simulink model "hcu_main_dspace"  (Simulink 8.2)
settings: Solver=FixedStepDiscrete  StartTime=0.0  StopTime=Inf  FixedStep=0.005  RelTol=1e-3
PostLoadFcn:
  | , if any(exist('dsrtsu_mdlpostloadfcn', 'file') == [2, 3, 6]), try dsrtsu_mdlpostloadfcn('Execute', bdroot); catch fprintf('Error in PostLoadFcn (dsrtsu_mdlpostloadfcn) for model "%s":\n %s\n', bdroot, lasterr); end, end,
values from neighbouring files (symbols this model uses):
  C_TASK_5MS_S = (	C_TICK_TIME_S      	)    [hcu_local_hdr.m]
  ENUM_GEARPOSN_1ST = uint8(  1  )    [hcu_local_hdr.m]
  ENUM_GEARPOSN_2ND = uint8(  2  )    [hcu_local_hdr.m]
  ENUM_GEARPOSN_3RD = uint8(  3  )    [hcu_local_hdr.m]
  ENUM_GEARPOSN_4TH = uint8(  4  )    [hcu_local_hdr.m]
  ENUM_GEARPOSN_5TH = uint8(  5  )    [hcu_local_hdr.m]
  ENUM_GEARPOSN_6TH = uint8(  6  )    [hcu_local_hdr.m]
  ENUM_GEARPOSN_R = uint8(  7  )    [hcu_local_hdr.m]
undefined symbols (not defined in the file or in its folder): rticanmm_blockfcn, rticanmm_initfcn
libraries: rtimmsu_dsrtlib x3, simulink x2, hal x2, app x1, rtiethernetudplib x1, inp x1, outp x1, hcu_lib x1
(part 1 of 4)
settings Model: DSRTSU_INTERNAL_RTI_VER=440  DSRTSU_INTERNAL_RTI_TYPE=rti1401  RTICANMMDATA=struct('GeneralSetupData',struct('modelroot','D:\ActiveSafetyDepartment\SVN\trunk\ADAS_Softwares\HTDragon\software\sw_development\arch','generalsettings',struct('filesettings',struct('destfolder',struct('Name','..\build\RTICANMM_FILES','Check',1),'buildfolder',struct('Name','.','Check',1),'AbsDestfolder',struct('Name','D:\ActiveSafetyDepartment\SVN\trunk\ADAS_Softwares\HTDragon\software\sw_development\build\RTICANMM_FILES'),'AbsBuildfolder',struct('Name','D:\ActiveSafetyDepartment\SVN\trunk\ADAS_Softwares\HTDragon\software\sw_development\arch'))),'options',struct('addpaths',1,'rmpaths',1,'addtrcexclusion',1,'cannavigator',struct('checkmonitoring',1),'show_usrtrc',0,'use_usrtrc',0,'addpath2usrmk',1),'advanced',struct('options',[1 1 1 1 1 1 1 1 1 1 1 1 1 1 1 1 1 1 1 1 1 1 1 1 1 1 1 1 1 1 1 1 1 1 1 1 1 1 1 1 1 1 1 1 1 1 1 1 1 1 1 1 1 1 1 1 1 1 1 1 1 1 1 1 1 1 1 1 1 1 1 1 1 1 1 1 1 1 1 1 1 1 1 1 1 1 1 1 1 1 1 1 1 1 1 1 1 1 1 1]),'MPSetup',{{}},'modelname','hcu_main_dspace','blockdata',struct('generalsettings',struct('filesettings',struct('destfolder',struct('Name','.','Check',1),'AbsDestfolder',struct('Name','T:\TOOL_SOURCES\CANnedy\m'),'buildfolder',struct('Name','.','Check',1),'AbsBuildfolder',struct('Name','C:\MATLAB6p5\work'))),'options',struct('addpaths',1,'rmpaths',1,'addpath2usrmk',1),'modelname','rticanmmlib','modelroot','T:\TOOL_SOURCES\CANnedy\m'),'MMType','RTICANMM','block',['hcu_main_dspace/RTICANMM' char(10) 'GeneralSetup'],'userdata',struct('HostServiceChannelID',{{'CAN_2',[],'CAN_1'}}),'RTI',struct('Type','RTI1401','Ver','7.2','Date','02-May-2014'),'version','3.0.735671.4434490741'))  DSRTSU_INTERNAL_RTIFPGA=30  Creator=11116  LastModifiedBy=14069  BufferReuse=off
settings DataIOCC: SignalLoggingSaveFormat=Dataset
settings OptimizationCC: BlockReduction=off  OptimizeBlockIOStorage=off  BufferReuse=off  ExpressionFolding=off  ExpressionDepthLimit=128  LocalBlockOutputs=off
settings DebuggingCC: CheckSSInitialOutputMsg=off  FcnCallInpInsideContextMsg=EnableAllAsError  StateNameClashWarn=none
settings HardwareCC: ProdIntDivRoundTo=Zero  ProdEndianess=BigEndian  ProdHWDeviceType=Generic->Custom  TargetIntDivRoundTo=Zero  TargetEndianess=BigEndian  TargetHWDeviceType=Generic->Custom
settings RTWCC: SystemTargetFile=rti1401.tlc  MakeCommand=make_rti  TemplateMakefile=rti1401.tmf  Description=dSPACE DS1401 Hardware Platform  ProcessScript=rti1401_make_rtw_hook
settings STFCustomTargetCC: CodeReplacementLibrary=ANSI_C  ParMdlRefBuildCompliant=on  GeneratePreprocessorConditionals=Disable all  SystemTargetFile=rti1401.tlc
settings GRTTargetCC: CompOptLevelCompliant=off  ConcurrentExecutionCompliant=off  MatFileLogging=off  ExtModeMexFile=noextcomm
settings CustomProperty: DataType=RTWOptions_EnumType_C__Program Files (x86)_dSPACE RCPHIL 2014-A_MATLAB_RTI_RTI1401_TLC_rti1401_1InitialSimState  Value=RUN
settings EnumStrPairs: String=RUN

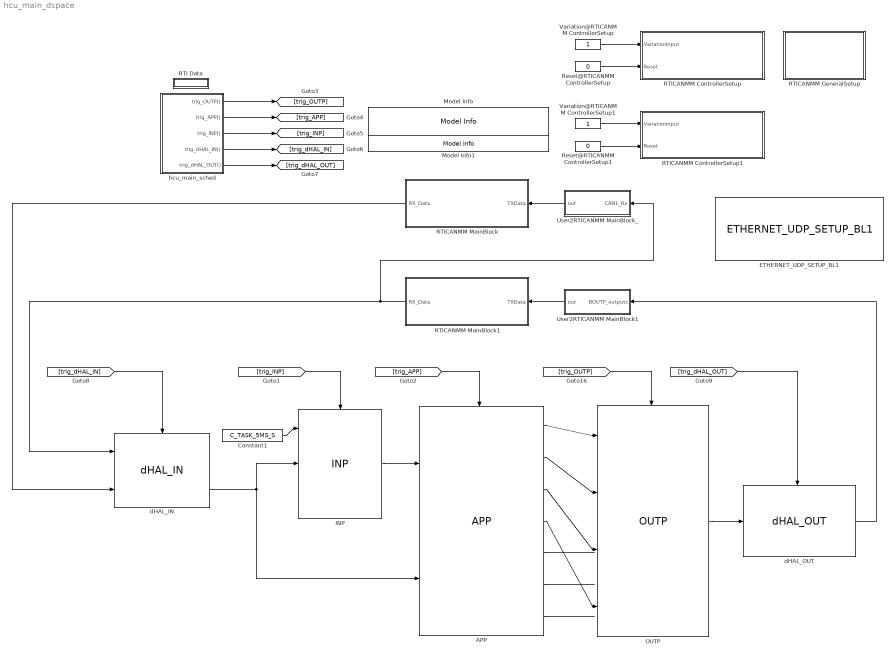
== system hcu_main_dspace ==
  APP : app/APP
  Constant1 : Constant  Value=C_TASK_5MS_S  OutDataTypeStr=single
  ETHERNET_UDP_SETUP_BL1 : rtiethernetudplib/ETHERNET_UDP_SETUP_BL1  DSProperties=struct('RTI',struct('Version',uint32(1),'BlockType',struct('isSLSource',uint8(0),'isSLSink',uint8(0),'isHWSource',uint8(0),'isHWSink',uint8(0),'isSetup',uint8(0),'isInline',uint8(1),'isNonInline',uint8(1),'isInterrupt',uint8(0),'isChannelwise',uint8(0)),'IOBoardType','DSETHERNETUDP','UnitType','ETHUDP','Identifier','SETUP','DialogType','ML','BlockSet','RTIETHERNETUDP','SlaveProcessor','NONE'))  RTIBlockInterface=struct('OutputPortsActive',0,'OutputPortsWidth',int32(1),'DialogFcn','rtiethernetudpsetupgui','InitLevel',3,'BlockDisplay',{{['Ethernet UDP Setup\nInterface Name: rti_ethernet_interface_name\nBoard Type: ETH Type 1\nModule: 1\nLocal IP Address: 192.168.140.11'],'center'}},'IconTransparency','on','BlockName',struct('Token',{{'ETHERNET_UDP_SETUP_BL1'}}))  RTIBlockParameters=struct('BoardType',{{1,'OFF',[]}},'ModuleNo',{{1,'ON',[1 16]}},'ChannelNo',{{1,'ON',[1 2]}},'InterfaceName',{{'rti_ethernet_interface_name','OFF',[]}},'LocalIpAddress',{{'192.168.140.11','OFF',[]}},'EnableSocket1',{{1,'OFF',[0 1]}},'LocalPortSocket1',{{'30000','OFF',[0 65535]}},'RemoteIpAddrSocket1',{{'192.168.140.10','OFF',[]}},'RemotePortSocket1',{{'30000','OFF',[0 65535]}},'EnableSocket2',{{1,'OFF',[0 1]}},'LocalPortSocket2',{{'30000','OFF',[0 65535]}},'RemoteIpAddrSocket2',{{'0.0.0.0','OFF',[]}},'RemotePortSocket2',{{'0','OFF',[0 65535]}},'EnableSocket3',{{0,'OFF',[0 1]}},'LocalPortSocket3',{{'5002','OFF',[0 65535]}},'RemoteIpAddrSocket3',{{'XXX.XXX.XXX.XXX','OFF',[]}},'RemotePortSocket3',{{'5002','OFF',[0 65535]}},'EnableSocket4',{{0,'OFF',[0 1]}},'LocalPortSocket4',{{'5003','OFF',[0 65535]}},'RemoteIpAddrSocket4',{{'XXX.XXX.XXX.XXX','OFF',[]}},'RemotePortSocket4',{{'5003','OFF',[0 65535]}},'LocalIpAddrHex',{{3232271371,'OFF',[]}},'RemoteIpAddrSocket1Hex',{{3232271370,'OFF',[]}},'RemoteIpAddrSocket2Hex',{{0,'OFF',[]}},'RemoteIpAddrSocket3Hex',{{0,'OFF',[]}},'RemoteIpAddrSocket4Hex',{{0,'OFF',[]}})  RTISFcnParameters=struct('BoardType','double','ModuleNo','double','ChannelNo','double','InterfaceName','char','LocalIpAddress','char','EnableSocket1','double','LocalPortSocket1','double','RemoteIpAddrSocket1','char','RemotePortSocket1','double','EnableSocket2','double','LocalPortSocket2','double','RemoteIpAddrSocket2','char','RemotePortSocket2','double','EnableSocket3','double','LocalPortSocket3','double','RemoteIpAddrSocket3','char','RemotePortSocket3','double','EnableSocket4','double','LocalPortSocket4','double','RemoteIpAddrSocket4','char','RemotePortSocket4','double','LocalIpAddrHex','double','RemoteIpAddrSocket1Hex','double','RemoteIpAddrSocket2Hex','double','RemoteIpAddrSocket3Hex','double','RemoteIpAddrSocket4Hex','double')  RTIBlockParaDefault=struct('BoardType',1,'ModuleNo',1,'ChannelNo',1,'InterfaceName','rti_ethernet_interface_name','LocalIpAddress','XXX.XXX.XXX.XXX','EnableSocket1',0,'LocalPortSocket1',5000,'RemoteIpAddrSocket1','XXX.XXX.XXX.XXX','RemotePortSocket1',5000,'EnableSocket2',0,'LocalPortSocket2',5001,'RemoteIpAddrSocket2','XXX.XXX.XXX.XXX','RemotePortSocket2',5001,'EnableSocket3',0,'LocalPortSocket3',5002,'RemoteIpAddrSocket3','XXX.XXX.XXX.XXX','RemotePortSocket3',5002,'EnableSocket4',0,'LocalPortSocket4',5003,'RemoteIpAddrSocket4','XXX.XXX.XXX.XXX','RemotePortSocket4',5003,'LocalIpAddrHex',0,'RemoteIpAddrSocket1Hex',0,'RemoteIpAddrSocket2Hex',0,'RemoteIpAddrSocket3Hex',0,'RemoteIpAddrSocket4Hex',0)
  INP : inp/INP
  Model Info : simulink/Model-Wide Utilities/Model Info  InitialBlockCM=None  BlockCM=None  Frame=off  DisplayStringWithTags=%<ModelName>  HorizontalTextAlignment=Center  LeftAlignmentValue=0.5  SourceBlockDiagram=hcu_main_dspace  TagMaxNumber=20
  Model Info1 : simulink/Model-Wide Utilities/Model Info  InitialBlockCM=None  BlockCM=None  Frame=off  DisplayStringWithTags=$Id: ADAS_Test.slx 244 2013-12-20 03:05:12Z JuneXmas $  HorizontalTextAlignment=Center  LeftAlignmentValue=0.5  SourceBlockDiagram=hcu_main_dspace  TagMaxNumber=20
  OUTP : outp/OUTP
  RTI Data : Subsystem  Tag=struct('RTIDataServer',struct('RTIDataServerVs','2','RTIModelDescription','struct(''main'',''hcu_main_dspace'',''sub'','''',''isMp'',0)'))  LoadFcn="if exist('rtidc'), try,  rtidc('DataHostBlockClbLoad', gcbh); catch, disp(['Warning: ''LoadFcn'' for RTI Data block failed: ' lasterr]); end, end,"  mask(RTI_DATA_HOST){}
      mask help:
      | RTI Data Block.
      | This block is used by RTI to store internal model-dependent data.
      | Please keep this block on the root level of the model. Deleting this block will result in data loss.
      |
      | NEVER DELETE OR COPY THIS BLOCK!
      settings: CopyFcn="if exist('rtidc'), try,  rtidc('DataHostBlockClbCopy', gcbh); catch, disp(['Warning: ''CopyFcn'' for RTI Data block failed: ' lasterr]); end, end,"  DeleteFcn="if exist('rtidc'), try,  rtidc('DataHostBlockClbDelete', gcbh); catch, disp(['Warning: ''DeleteFcn'' for RTI Data block failed: ' lasterr]); end, end,"  ModelCloseFcn="if exist('rtidc'), try,  rtidc('DataHostBlockClbModelClose', gcbh); catch, disp(['Warning: ''ModelCloseFcn'' for RTI Data block failed: ' lasterr]); end, end,"  PreSaveFcn="if exist('rtidc'), try,  rtidc('DataHostBlockClbPreSave', gcbh); catch, disp(['Warning: ''PreSaveFcn'' for RTI Data block failed: ' lasterr]); end, end,"  PostSaveFcn="if exist('rtidc'), try,  rtidc('DataHostBlockClbPostSave', gcbh); catch, disp(['Warning: ''PostSaveFcn'' for RTI Data block failed: ' lasterr]); end, end,"  NameChangeFcn="if exist('rtidc'), try,  rtidc('DataHostBlockClbNameChange', gcbh); catch, disp(['Warning: ''NameChangeFcn'' for RTI Data block failed: ' lasterr]); end, end,"
      mask Help:
      | RTI Data Block.
      | This block is used by RTI to store internal model-dependent data.
      | Please keep this block on the root level of the model. Deleting this block will result in data loss.
      | 
      | NEVER DELETE OR COPY THIS BLOCK!
      mask Display:
      | text(0.5, 0.5, 'RTI Data', 'HorizontalAlignment', 'center');
      | plot([1 0]);
  RTICANMM ControllerSetup : Subsystem  InitFcn=rticanmm_blockfcn('InitFcn', 'CANnedySetup', gcb)  ClipboardFcn=rticanmm_blockfcn('ClipboardFcn', 'CANnedySetup', gcb)  mask(RTICANMM){DSProperties=struct('RTI',struct('Version',uint32(1),'BlockType',struct('isSLSource',uint8(1),'isSLSink',uint8(1),'isHWSource',uint8(0),'isHWSink',uint8(0),'isSetup',uint8(0),'isInline',uint8(1),'isNonInline',uint8(0),'isInterrupt',uint8(0),'isChannelwise',uint8(0)),'IOBoardType','RTICANMM','UnitType','RTICANMM','Identifier','BUSSETUP','DialogType','SL','BlockSet','RTICANMM','SlaveProcessor','CAN')), CANMMProperties=struct('cannedy',struct('data',struct('options',struct('controllername','CAN_1','controllernameautomatic',[],'loglevel','0','checkrealtime',0,'checkchangebaudrate',0,'sampletime','1.000','CANControllerStatus',0,'NumberofStuffErr',0,'NumberofFormErr',0,'NumberofAckErr',0,'NumberofBit0Err',0,'NumberofsuccrecRX',0,'Numberofsuccsent',0,'NumberofBit1Err',0,'NumberofCRCErr',0,'NumberoflostRX',0,'Busoff',0,'Busload',0,'OperationPending',0,'TxRetryCount',3,'addtrcexclusion',logical(1),'cannavigator',struct('checkmonitoring',0,'checkinternmonitoring',0),'show_usrtrc',0,'use_usrtrc',0),'modelroot','D:\ADAS\ADAS\trunk\Demo\AI\ACM_d2','generalsettings',struct('setupdata',struct('board',['CAN Type 1'],'boardno',1,'channelno',1,'Type','STD','transceiver','ISO11898-2','busconfig','0x0','feedthrough','false','resistance',struct('r120',0,'roff',1,'r16',1,'r10',0),'baudrate','500','Frequency',[24 36],'samplemode',1,'commChannelTJA1041',6,'config',struct('standard',1,'advanced',0,'register',struct('btr0','0xC0','btr1','0x6F','sp','70','sjw','3','tseg1','15','tseg2','6','brp','0','smpl','0','btr0_36','0x41','btr1_36','0x1E','sp_36','88','sjw_36','1','tseg1_36','14','tseg2_36','1','brp_36','1','smpl_36','0','btr0_64','0x43','btr1_64','0x1C','sp_64','87','sjw_64','1','tseg1_64','12','tseg2_64','1','brp_64','3','smpl_64','0')),'channelcfg',struct('INTENDISABLE','CAN_INT_DISABLE','intenable',0),'SETUPID','RTICANMM_CAN_1_ID','CONTROLLER_ID','CANMM_CTL_SETUP_CAN_1','mainblock_includefile','RTICANMM_SETUP_CAN_1','termination','TERMINATION_OFF'),'filesettings',struct('destfolder',struct('Name','RTICANMM_FILES','Check',1),'buildfolder',struct('Name','.','Check',1))),'advanced',struct('options',[1 1 1 1 1 1 1 1 1 1 1 1 1 1 1 1 1 1 1 1 1 1 1 1 1 1 1 1 1 1 1 1 1 1 1 1 1 1 1 1 1 1 1 1 1 1 1 1 1 1 1 1 1 1 1 1 1 1 1 1 1 1 1 1 1 1 1 1 1 1 1 1 1 1 1 1 1 1 1 1 1 1 1 1 1 1 1 1 1 1 1 1 1 1 1 1 1 1 1 1]),'partialnetdata',struct('switchedon',0,'format','STD','idmask',['XXXXX XXXXXXXX XXXXXXXX XXXXXXXX'],'idcode','0','idfilter','0','datamaskused',0,'datalength','0','datamask','0x0000000000000000','partialnetworkenable',0)),'blk',['hcu_main_dspace/RTICANMM' char(10) 'ControllerSetup'],'allgeneratedfiles',{{'D:\ActiveSafetyDepartment\SVN\trunk\ADAS_Softwares\HTDragon\software\sw_development\build\RTICANMM_FILES\RTICANMM_SETUP_CAN_1.c','D:\ActiveSafetyDepartment\SVN\trunk\ADAS_Softwares\HTDragon\software\sw_development\build\RTICANMM_FILES\RTICANMM_SETUP_CAN_1.h','d:\activesafetydepartment\svn\trunk\adas_softwares\htdragon\software\sw_development\build\rticanmm_files\rticanmm_setup_can_1.mexw32'}},'ismp',logical(0),'BlockDataVersion','0.6.0','recreate',0,'CANnedyTag','EPAS'),'CANnedynew',0,'CANnedySettings','CAN_1','GeneratedFiles',{{'D:\ActiveSafetyDepartment\SVN\trunk\ADAS_Softwares\HTDragon\software\sw_development\build\RTICANMM_FILES\RTICANMM_SETUP_CAN_1.c','D:\ActiveSafetyDepartment\SVN\trunk\ADAS_Softwares\HTDragon\software\sw_development\build\RTICANMM_FILES\RTICANMM_SETUP_CAN_1.h','d:\activesafetydepartment\svn\trunk\adas_softwares\htdragon\software\sw_development\build\rticanmm_files\rticanmm_setup_can_1.mexw32'}},'SFCN','RTICANMM_SETUP_CAN_1.c','HostService',struct('Tags',struct('DATA','RTICANMM_MonitorData','Enable','CANMMMonitor_CAN_1','TimeStamp','MonitoringTimeStamp_CAN_1'),'DATA',struct('Length',4),'Info',struct('Desc',{'ID','Service','Data1','Data2'}),'Names',struct('Enable','Monitoring_Enable','TimeStamp','Monitoring_TimeStamp'),'ChannelID',3)), CANMMType=CANnedySetup, CANMMFolder=D:\ActiveSafetyDepartment\SVN\trunk\ADAS_Softwares\HTDragon\software\sw_development\arch, CANMMDestFolder=..\build\RTICANMM_FILES, CANMMSettings=CAN_1, CANMMSFcn=RTICANMM_SETUP_CAN_1, CANMMBoard=DS1401, CANMMBoardNum=1, CANMMChannel=1}
      settings: AttributesFormatString=%<CANMMSettings>: %<CANMMBoard>_B%<CANMMBoardNum>_C%<CANMMChannel>  CopyFcn=rticanmm_blockfcn('CopyFcn', 'CANnedySetup', gcb)  DeleteFcn=rticanmm_blockfcn('DeleteFcn', 'CANnedySetup', gcb)  ModelCloseFcn=rticanmm_blockfcn('ModelCloseFcn', 'CANnedySetup', gcb)  NameChangeFcn=rticanmm_blockfcn('NameChangeFcn', 'CANnedySetup', gcb)  OpenFcn=try, rticanmm_setup_gui('create',gcb); ; catch,errordlg({lasterr, '','Please check your RTI installation.'},['Error: ' upper(bdroot)], 'replace'); end  MoveFcn=rticanmm_blockfcn('MoveFcn', 'CANnedySetup', gcb)
      mask Help: eval('rticanmm_quickstart(''create'', gcb);', 'disp(lasterr);')
      mask Display:
      | disp('RTI CAN\nMultiMessage\nControllerSetup')
      | 
      | port_label('input', 1 , 'Variation')
      | port_label('input', 2 , 'Reset')
  RTICANMM ControllerSetup1 : Subsystem  InitFcn=rticanmm_blockfcn('InitFcn', 'CANnedySetup', gcb)  ClipboardFcn=rticanmm_blockfcn('ClipboardFcn', 'CANnedySetup', gcb)  mask(RTICANMM){DSProperties=struct('RTI',struct('Version',uint32(1),'BlockType',struct('isSLSource',uint8(1),'isSLSink',uint8(1),'isHWSource',uint8(0),'isHWSink',uint8(0),'isSetup',uint8(0),'isInline',uint8(1),'isNonInline',uint8(0),'isInterrupt',uint8(0),'isChannelwise',uint8(0)),'IOBoardType','RTICANMM','UnitType','RTICANMM','Identifier','BUSSETUP','DialogType','SL','BlockSet','RTICANMM','SlaveProcessor','CAN')), CANMMProperties=struct('cannedy',struct('data',struct('options',struct('controllername','CAN_2','controllernameautomatic',[],'loglevel','0','checkrealtime',0,'checkchangebaudrate',0,'sampletime','1.000','CANControllerStatus',0,'NumberofStuffErr',0,'NumberofFormErr',0,'NumberofAckErr',0,'NumberofBit0Err',0,'NumberofsuccrecRX',0,'Numberofsuccsent',0,'NumberofBit1Err',0,'NumberofCRCErr',0,'NumberoflostRX',0,'Busoff',0,'Busload',0,'OperationPending',0,'TxRetryCount',3,'addtrcexclusion',logical(1),'cannavigator',struct('checkmonitoring',0,'checkinternmonitoring',0),'show_usrtrc',0,'use_usrtrc',0),'modelroot','D:\ActiveSafetyDepartment\SVN\trunk\Demo\AI\ACM_d5','generalsettings',struct('setupdata',struct('board',['CAN Type 1'],'boardno',1,'channelno',2,'Type','STD','transceiver','ISO11898-2','busconfig','0x0','feedthrough','false','resistance',struct('r120',1,'roff',0,'r16',1,'r10',0),'baudrate','500','Frequency',[24 36],'samplemode',1,'commChannelTJA1041',6,'config',struct('standard',1,'advanced',0,'register',struct('btr0','0xC0','btr1','0x6F','sp','70','sjw','3','tseg1','15','tseg2','6','brp','0','smpl','0','btr0_36','0x41','btr1_36','0x1E','sp_36','88','sjw_36','1','tseg1_36','14','tseg2_36','1','brp_36','1','smpl_36','0','btr0_64','0x43','btr1_64','0x1C','sp_64','87','sjw_64','1','tseg1_64','12','tseg2_64','1','brp_64','3','smpl_64','0')),'channelcfg',struct('INTENDISABLE','CAN_INT_DISABLE','intenable',0),'SETUPID','RTICANMM_CAN_2_ID','CONTROLLER_ID','CANMM_CTL_SETUP_CAN_2','mainblock_includefile','RTICANMM_SETUP_CAN_2','termination','TERMINATION_ON'),'filesettings',struct('destfolder',struct('Name','RTICANMM_FILES','Check',1),'buildfolder',struct('Name','.','Check',1))),'advanced',struct('options',[1 1 1 1 1 1 1 1 1 1 1 1 1 1 1 1 1 1 1 1 1 1 1 1 1 1 1 1 1 1 1 1 1 1 1 1 1 1 1 1 1 1 1 1 1 1 1 1 1 1 1 1 1 1 1 1 1 1 1 1 1 1 1 1 1 1 1 1 1 1 1 1 1 1 1 1 1 1 1 1 1 1 1 1 1 1 1 1 1 1 1 1 1 1 1 1 1 1 1 1]),'partialnetdata',struct('switchedon',0,'format','STD','idmask',['XXXXX XXXXXXXX XXXXXXXX XXXXXXXX'],'idcode','0','idfilter','0','datamaskused',0,'datalength','0','datamask','0x0000000000000000','partialnetworkenable',0)),'blk',['hcu_main_dspace/RTICANMM' char(10) 'ControllerSetup1'],'allgeneratedfiles',{{'D:\ActiveSafetyDepartment\SVN\trunk\ADAS_Softwares\HTDragon\software\sw_development\build\RTICANMM_FILES\RTICANMM_SETUP_CAN_2.c','D:\ActiveSafetyDepartment\SVN\trunk\ADAS_Softwares\HTDragon\software\sw_development\build\RTICANMM_FILES\RTICANMM_SETUP_CAN_2.h','d:\activesafetydepartment\svn\trunk\adas_softwares\htdragon\software\sw_development\build\rticanmm_files\rticanmm_setup_can_2.mexw32'}},'ismp',logical(0),'BlockDataVersion','0.6.0','recreate',0,'CANnedyTag','TEST'),'CANnedynew',0,'CANnedySettings','CAN_2','GeneratedFiles',{{'D:\ActiveSafetyDepartment\SVN\trunk\ADAS_Softwares\HTDragon\software\sw_development\build\RTICANMM_FILES\RTICANMM_SETUP_CAN_2.c','D:\ActiveSafetyDepartment\SVN\trunk\ADAS_Softwares\HTDragon\software\sw_development\build\RTICANMM_FILES\RTICANMM_SETUP_CAN_2.h','d:\activesafetydepartment\svn\trunk\adas_softwares\htdragon\software\sw_development\build\rticanmm_files\rticanmm_setup_can_2.mexw32'}},'SFCN','RTICANMM_SETUP_CAN_2.c','HostService',struct('Tags',struct('DATA','RTICANMM_MonitorData','Enable','CANMMMonitor_CAN_2','TimeStamp','MonitoringTimeStamp_CAN_2'),'DATA',struct('Length',4),'Info',struct('Desc',{'ID','Service','Data1','Data2'}),'Names',struct('Enable','Monitoring_Enable','TimeStamp','Monitoring_TimeStamp'),'ChannelID',1)), CANMMType=CANnedySetup, CANMMFolder=D:\ActiveSafetyDepartment\SVN\trunk\ADAS_Softwares\HTDragon\software\sw_development\arch, CANMMDestFolder=..\build\RTICANMM_FILES, CANMMSettings=CAN_2, CANMMSFcn=RTICANMM_SETUP_CAN_2, CANMMBoard=DS1401, CANMMBoardNum=1, CANMMChannel=2}
      settings: AttributesFormatString=%<CANMMSettings>: %<CANMMBoard>_B%<CANMMBoardNum>_C%<CANMMChannel>  CopyFcn=rticanmm_blockfcn('CopyFcn', 'CANnedySetup', gcb)  DeleteFcn=rticanmm_blockfcn('DeleteFcn', 'CANnedySetup', gcb)  ModelCloseFcn=rticanmm_blockfcn('ModelCloseFcn', 'CANnedySetup', gcb)  NameChangeFcn=rticanmm_blockfcn('NameChangeFcn', 'CANnedySetup', gcb)  OpenFcn=try, rticanmm_setup_gui('create',gcb); ; catch,errordlg({lasterr, '','Please check your RTI installation.'},['Error: ' upper(bdroot)], 'replace'); end  MoveFcn=rticanmm_blockfcn('MoveFcn', 'CANnedySetup', gcb)
      mask Help: eval('rticanmm_quickstart(''create'', gcb);', 'disp(lasterr);')
      mask Display:
      | disp('RTI CAN\nMultiMessage\nControllerSetup')
      | 
      | port_label('input', 1 , 'Variation')
      | port_label('input', 2 , 'Reset')
  RTICANMM GeneralSetup : Subsystem  InitFcn=rticanmm_initfcn(gcb, 'CANnedySettings')  ClipboardFcn=rticanmm_blockfcn('ClipboardFcn', 'CANnedySettings', gcb)  mask(RTICANMM){DSProperties=struct('RTI',struct('Version',uint32(1),'BlockType',struct('isSLSource',uint8(1),'isSLSink',uint8(1),'isHWSource',uint8(0),'isHWSink',uint8(0),'isSetup',uint8(0),'isInline',uint8(1),'isNonInline',uint8(0),'isInterrupt',uint8(0),'isChannelwise',uint8(0)),'IOBoardType','RTICANMM','UnitType','RTICANMM','Identifier','GENERALSETUP','DialogType','SL','BlockSet','RTICANMM','SlaveProcessor','CAN')), CANMMDestFolder=..\build\RTICANMM_FILES, CANMMBuildDir=., CANMMAddPaths=on, CANMMAddpathUserMake=on, CANMMRemovePathOnclose=on, CANMMType=CANnedySettings, CANMMProperties=struct('modelroot','D:\ActiveSafetyDepartment\SVN\trunk\ADAS_Softwares\HTDragon\software\sw_development\arch','generalsettings',struct('filesettings',struct('destfolder',struct('Name','..\build\RTICANMM_FILES','Check',1),'buildfolder',struct('Name','.','Check',1),'AbsDestfolder',struct('Name','D:\ActiveSafetyDepartment\SVN\trunk\ADAS_Softwares\HTDragon\software\sw_development\build\RTICANMM_FILES'),'AbsBuildfolder',struct('Name','D:\ActiveSafetyDepartment\SVN\trunk\ADAS_Softwares\HTDragon\software\sw_development\arch'))),'options',struct('addpaths',1,'rmpaths',1,'addtrcexclusion',1,'cannavigator',struct('checkmonitoring',1),'show_usrtrc',0,'use_usrtrc',0,'addpath2usrmk',1),'advanced',struct('options',[1 1 1 1 1 1 1 1 1 1 1 1 1 1 1 1 1 1 1 1 1 1 1 1 1 1 1 1 1 1 1 1 1 1 1 1 1 1 1 1 1 1 1 1 1 1 1 1 1 1 1 1 1 1 1 1 1 1 1 1 1 1 1 1 1 1 1 1 1 1 1 1 1 1 1 1 1 1 1 1 1 1 1 1 1 1 1 1 1 1 1 1 1 1 1 1 1 1 1 1]),'MPSetup',{{}},'modelname','hcu_main_dspace','blockdata',struct('generalsettings',struct('filesettings',struct('destfolder',struct('Name','.','Check',1),'AbsDestfolder',struct('Name','T:\TOOL_SOURCES\CANnedy\m'),'buildfolder',struct('Name','.','Check',1),'AbsBuildfolder',struct('Name','C:\MATLAB6p5\work'))),'options',struct('addpaths',1,'rmpaths',1,'addpath2usrmk',1),'modelname','rticanmmlib','modelroot','T:\TOOL_SOURCES\CANnedy\m'),'MMType','RTICANMM','block',['hcu_main_dspace/RTICANMM' char(10) 'GeneralSetup'],'userdata',struct('HostServiceChannelID',{{'CAN_2',[],'CAN_1'}}),'RTI',struct('Type','RTI1401','Ver','7.2','Date','02-May-2014'),'version','3.0.735671.4434490741')}
      mask prompts: CANMMDestFolder "Destination Folder for generated Files:"; CANMMBuildDir "Build Directory (*_usr.mk, *_usr.trc)"; CANMMAddPaths "Add Paths automatically"; CANMMAddpathUserMake "Add Paths to UserMake-File"; CANMMRemovePathOnclose "Remove added Path on ModelClose"
      mask init:
      | rticanmm_initfcn(gcb,'CANnedyGeneralSettings')
      settings: CopyFcn=rticanmm_blockfcn('CopyFcn', 'CANnedySettings', gcb)  DeleteFcn=rticanmm_blockfcn('DeleteFcn', 'CANnedySettings', gcb)  ModelCloseFcn=rticanmm_blockfcn('CloseFcn', 'CANnedyGeneralSettings', gcb)  NameChangeFcn=rticanmm_blockfcn('NameChangeFcn', 'CANnedySettings', gcb)  OpenFcn=try, rticanmm_gs_gui('create',gcb), ; catch,errordlg({lasterr, '','Please check your RTI installation.'},['Error: ' upper(bdroot)], 'replace'); end  MoveFcn=rticanmm_blockfcn('MoveFcn', 'CANnedySettings', gcb)
      mask Help: eval('rticanmm_quickstart(''create'', gcb);', 'disp(lasterr);')
      mask Display: disp(sprintf(['RTI CAN\nMultiMessage\nGeneralSetup']))
  RTICANMM MainBlock : Subsystem  InitFcn=rticanmm_blockfcn('InitFcn', 'CANnedy', gcb)  ClipboardFcn=rticanmm_blockfcn('ClipboardFcn', 'CANnedy', gcb)  mask(RTICANMM){DSProperties=struct('RTI',struct('Version',uint32(1),'BlockType',struct('isSLSource',uint8(1),'isSLSink',uint8(1),'isHWSource',uint8(0),'isHWSink',uint8(0),'isSetup',uint8(0),'isInline',uint8(1),'isNonInline',uint8(0),'isInterrupt',uint8(0),'isChannelwise',uint8(0)),'IOBoardType','RTICANMM','UnitType','RTICANMM','Identifier','Mainblock','DialogType','SL','BlockSet','RTICANMM','SlaveProcessor','CAN')), CANMMProperties=struct('RTICANMMVersion','3.0','RTICANMMVersionIntern','3.0.735671.4434490741','RTICANMMDate','02-May-2014','Settings','RTICANMM_MAIN_CAN_2','UserTracePath','','ModelPath','D:\ActiveSafetyDepartment\SVN\trunk\ADAS_Softwares\HTDragon\software\sw_development\arch','filesettings',struct('FileName','..\..\..\..\CAN\IDIADA_CAN2_Chimo.dbc','IsRelative',1,'ClusterId',1,'ClusterList',{{'default'}},'destfolder',struct('Name','..\build\RTICANMM_FILES','Check',1),'buildfolder',struct('Name','.','Check',1),'onlyfreerawcapture',0,'overlapping2variant',0),'onlyfreerawcapture',0,'Board',['CAN Type 1'],'BoardNum','1','ChannelNum','2','Variation','1','SetupId','CAN_2','MARK',['2DBE3E4EF1BAADAF8427111C40D4CA';'085B5D53DE150542DA650E691DA8DD';'A43ABF07D72688DDE05877E4A4CD4F';'3C583CAA49F93CC5669B070848561E';'93657246D29663F85A60CA3CB29854'],'date','03-Dec-2015','clock',['03.12.2015 15:57:37'],'recreate',0,'RTIVER','RTI1401','j1939',0,'TRC',struct('include',1),'rtsupport',struct('XMLFile','D:\ActiveSafetyDepartment\SVN\trunk\ADAS_Softwares\HTDragon\software\sw_development\build\RTICANMM_FILES\RTICANMM_MAIN_CAN_2.xml','DBCXML',struct('Path','D:\ActiveSafetyDepartment\SVN\trunk\ADAS_Softwares\HTDragon\software\sw_development\build\RTICANMM_FILES\RTICANMM_MAIN_CAN_2_dbc.xml','support',1,'Name','IDIADA_CAN2_Chimo.dbc','Date',['15-十月-2015 11:52:08'],'Type','standard','DBCSupport','ON'))), CANMMType=CANnedy, CANMMUserTraceMerged=off, CANMMUserTracePath=, CANMMChannelNum=2, CANMMBoardNum=1, CANMMDestFolder=..\build\RTICANMM_FILES, CANMMFolder=., CANMMSetupId=CAN_2, CANMMsave2mat=['2DBE3E4EF1BAADAF8427111C40D4CA';'085B5D53DE150542DA650E691DA8DD';'A43ABF07D72688DDE05877E4A4CD4F';'3C583CAA49F93CC5669B070848561E';'93657246D29663F85A60CA3CB29854'], CANMMName=CAN_2, CANMMSettings=RTICANMM_MAIN_CAN_2, CANMMIntermediateTag=RTICANMM_MAIN_CAN_2_intermediate, CANMMsfcnname=RTICANMM_MAIN_CAN_2}
      mask init:
      | rticanmm_initfcn(gcb, CANMMType, CANMMsfcnname)
      settings: AttributesFormatString=CAN_2[CAN_2]: DS1401_B1_C2_V1  CopyFcn=rticanmm_blockfcn('CopyFcn', 'CANnedy', gcb)  DeleteFcn=rticanmm_blockfcn('DeleteFcn', 'CANnedy', gcb)  ModelCloseFcn=rticanmm_blockfcn('ModelCloseFcn', 'CANnedy', gcb)  NameChangeFcn=rticanmm_blockfcn('NameChangeFcn', 'CANnedy', gcb)  OpenFcn=try, rticanmm_main_gui('create',gcb); ; catch,errordlg({lasterr, '','Please check your RTI installation.'},['Error: ' upper(bdroot)], 'replace'); end  MoveFcn=rticanmm_blockfcn('MoveFcn', 'CANnedy', gcb)
      mask Help: eval('rticanmm_quickstart(''create'', gcb);', 'disp(lasterr);')
      mask Display:
      | disp(sprintf('RTI CAN\nMultiMessage\nMainSetup'))
      | port_label('input', 1, 'TX Data')
      | port_label('output', 1, 'RX Data')
  RTICANMM MainBlock1 : Subsystem  InitFcn=rticanmm_blockfcn('InitFcn', 'CANnedy', gcb)  ClipboardFcn=rticanmm_blockfcn('ClipboardFcn', 'CANnedy', gcb)  mask(RTICANMM){DSProperties=struct('RTI',struct('Version',uint32(1),'BlockType',struct('isSLSource',uint8(1),'isSLSink',uint8(1),'isHWSource',uint8(0),'isHWSink',uint8(0),'isSetup',uint8(0),'isInline',uint8(1),'isNonInline',uint8(0),'isInterrupt',uint8(0),'isChannelwise',uint8(0)),'IOBoardType','RTICANMM','UnitType','RTICANMM','Identifier','Mainblock','DialogType','SL','BlockSet','RTICANMM','SlaveProcessor','CAN')), CANMMProperties=struct('RTICANMMVersion','3.0','RTICANMMVersionIntern','3.0.735671.4434490741','RTICANMMDate','02-May-2014','Settings','RTICANMM_MAIN_CAN_1','UserTracePath','','ModelPath','D:\ActiveSafetyDepartment\SVN\trunk\ADAS_Softwares\HTDragon\software\sw_development\arch','filesettings',struct('FileName','..\..\..\..\CAN\ADAS_CAN1_Mule1_BSGEMS_MVCU_MEPS_20150610_db.dbc','IsRelative',1,'ClusterId',1,'ClusterList',{{'default'}},'destfolder',struct('Name','..\build\RTICANMM_FILES','Check',1),'buildfolder',struct('Name','.','Check',1),'onlyfreerawcapture',0,'overlapping2variant',0),'onlyfreerawcapture',0,'Board',['CAN Type 1'],'BoardNum','1','ChannelNum','1','Variation','1','SetupId','CAN_1','MARK',['472D3A1A3D5208B3D30AB78F04E268';'A50162927E39700EACAFCCF6AEEB36';'6294BC9383410CB3E84E79B296AFCF';'84400670336E8CD48E57496AA42E44';'1090534234403A3283605A55A13471'],'date','03-Dec-2015','clock',['03.12.2015 15:58:16'],'recreate',0,'RTIVER','RTI1401','j1939',0,'TRC',struct('include',1),'rtsupport',struct('XMLFile','D:\ActiveSafetyDepartment\SVN\trunk\ADAS_Softwares\HTDragon\software\sw_development\build\RTICANMM_FILES\RTICANMM_MAIN_CAN_1.xml','DBCXML',struct('Path','D:\ActiveSafetyDepartment\SVN\trunk\ADAS_Softwares\HTDragon\software\sw_development\build\RTICANMM_FILES\RTICANMM_MAIN_CAN_1_dbc.xml','support',1,'Name','ADAS_CAN1_Mule1_BSGEMS_MVCU_MEPS_20150610_db.dbc','Date',['12-十一月-2015 09:30:54'],'Type','standard','DBCSupport','ON'))), CANMMType=CANnedy, CANMMUserTraceMerged=off, CANMMUserTracePath=, CANMMChannelNum=1, CANMMBoardNum=1, CANMMDestFolder=..\build\RTICANMM_FILES, CANMMFolder=., CANMMSetupId=CAN_1, CANMMsave2mat=['472D3A1A3D5208B3D30AB78F04E268';'A50162927E39700EACAFCCF6AEEB36';'6294BC9383410CB3E84E79B296AFCF';'84400670336E8CD48E57496AA42E44';'1090534234403A3283605A55A13471'], CANMMName=CAN_1, CANMMSettings=RTICANMM_MAIN_CAN_1, CANMMIntermediateTag=RTICANMM_MAIN_CAN_1_intermediate, CANMMsfcnname=RTICANMM_MAIN_CAN_1}
      mask init:
      | rticanmm_initfcn(gcb, CANMMType, CANMMsfcnname)
      settings: AttributesFormatString=CAN_1[CAN_1]: DS1401_B1_C1_V1  CopyFcn=rticanmm_blockfcn('CopyFcn', 'CANnedy', gcb)  DeleteFcn=rticanmm_blockfcn('DeleteFcn', 'CANnedy', gcb)  ModelCloseFcn=rticanmm_blockfcn('ModelCloseFcn', 'CANnedy', gcb)  NameChangeFcn=rticanmm_blockfcn('NameChangeFcn', 'CANnedy', gcb)  OpenFcn=try, rticanmm_main_gui('create',gcb); ; catch,errordlg({lasterr, '','Please check your RTI installation.'},['Error: ' upper(bdroot)], 'replace'); end  MoveFcn=rticanmm_blockfcn('MoveFcn', 'CANnedy', gcb)
      mask Help: eval('rticanmm_quickstart(''create'', gcb);', 'disp(lasterr);')
      mask Display:
      | disp(sprintf('RTI CAN\nMultiMessage\nMainSetup'))
      | port_label('input', 1, 'TX Data')
      | port_label('output', 1, 'RX Data')
  Reset@RTICANMM ControllerSetup : Constant  Value=0  OutDataTypeStr=boolean
  Reset@RTICANMM ControllerSetup1 : Constant  Value=0  OutDataTypeStr=boolean
  User2RTICANMM MainBlock1 : Subsystem
      mask Display: disp('Mapping\nto RTICANMM')
  User2RTICANMM MainBlock_ : Subsystem
      mask Display: disp('Mapping\nto RTICANMM')
  Variation@RTICANMM ControllerSetup : Constant  OutDataTypeStr=uint8
  Variation@RTICANMM ControllerSetup1 : Constant  OutDataTypeStr=uint8
  dHAL_IN : hal/dHAL_IN
  dHAL_OUT : hal/dHAL_OUT
  hcu_main_sched : Stateflow chart  TreatAsAtomicUnit=on
  wires:
  Variation@RTICANMM ControllerSetup/1 -> RTICANMM ControllerSetup/1(VariationInput)
  Reset@RTICANMM ControllerSetup/1 -> RTICANMM ControllerSetup/2(Reset)
  Variation@RTICANMM ControllerSetup1/1 -> RTICANMM ControllerSetup1/1(VariationInput)
  Reset@RTICANMM ControllerSetup1/1 -> RTICANMM ControllerSetup1/2(Reset)
  hcu_main_sched/1(trig_OUTP()) -> [trig_OUTP]
  hcu_main_sched/2(trig_APP()) -> [trig_APP]
  hcu_main_sched/3(trig_INP()) -> [trig_INP]
  [trig_INP] -> INP/Trigger
  [trig_OUTP] -> OUTP/Trigger
  [trig_APP] -> APP/Trigger
  INP/1 -> APP/1
  OUTP/1 -> dHAL_OUT/1
  Constant1/1 -> INP/1
  hcu_main_sched/4(trig_dHAL_IN()) -> [trig_dHAL_IN]
  [trig_dHAL_IN] -> dHAL_IN/Trigger
  [trig_dHAL_OUT] -> dHAL_OUT/Trigger
  APP/1 -> OUTP/1
  APP/2 -> OUTP/2
  APP/3 -> OUTP/3
  APP/4 -> OUTP/4
  APP/5 -> ?
  APP/6 -> ?
  APP/7 -> ?
  dHAL_IN/2 -> INP/2, APP/2
  User2RTICANMM MainBlock_/1(out) -> RTICANMM MainBlock/1(TXData)
  RTICANMM MainBlock1/1(RX_Data) -> dHAL_IN/1, User2RTICANMM MainBlock_/1(CAN1_Rx)
  hcu_main_sched/5(trig_dHAL_OUT()) -> [trig_dHAL_OUT]
  User2RTICANMM MainBlock1/1(out) -> RTICANMM MainBlock1/1(TXData)
  RTICANMM MainBlock/1(RX_Data) -> dHAL_IN/2
  dHAL_OUT/1 -> User2RTICANMM MainBlock1/1(BOUTP_outputs)

== system hcu_main_dspace/RTI Data ==
  RTI Data Store : Subsystem  Tag="struct('private',struct('version',struct('dsVer',uint32(2),'dsVerCreation',uint32(2),'RTI',struct('ver','7.1','type','RTI1401')),'access',struct('type','Model','isPerm',1,'created',['09-May-2014 08:49:11'],'modified',['04-Dec-2015 14:20:46'],'location','')),'public',struct('main',struct('data',[]),'sub',struct('name',{{'hcu_main_dspace'}},'data',{{struct('TH',struct('thTaskInfo',struct('taskType',{'TIMER','HWINT','TMRINT','SWINT','GLINT'},'tasksNumOf',{1,0,0,0,0},'srcIds',{{'TIMERA'},{},{},{},{}},'taskNames',{{['Timer Task 1']},{},{},{},{}})),'th_tc',struct('dataType','TASK','taskGroupId','','taskGroupList',{{}},'taskSchedulingPolicy','FCFS','taskType','TIMER','blkh',-1,'srcId','TIMERA','srcSgnName',['Timer A interrupt'],'srcCpuName','','taskName',['Timer Task 1  [0.005] s'],'taskNameDisplayExt','','smplTime',0.005,'smplTimeOffs',0,'hasFixedPriority',0,'priority',1,'hasFixedOvc',0,'ovcType',1,'ovcMax',1),'tc_th',struct('dataType','TASK','taskGroupId','','taskGroupList',{{}},'taskSchedulingPolicy','FCFS','taskType','TIMER','blkh',-1,'srcId','TIMERA','srcSgnName',['Timer A interrupt'],'srcCpuName','','taskName',['Timer Task 1  [0.005] s'],'taskNameDisplayExt','','smplTime',0.005,'smplTimeOffs',0,'hasFixedPriority',0,'priority',1,'hasFixedOvc',0,'ovcType',1,'ovcMax',1))}})))"  mask(RTI_DATA_STORE){}
      mask help:
      | RTI Data Store Block. This block is used by RTI to store internal model dependent data. Deleting this block will result in data loss.
      |
      | NEVER DELETE, COPY, OR MODIFY THIS BLOCK!
      mask Help:
      | RTI Data Store Block. This block is used by RTI to store internal model dependent data. Deleting this block will result in data loss.
      | 
      | NEVER DELETE, COPY, OR MODIFY THIS BLOCK!
      mask Display: text(0.5, 0.5, ' ', 'HorizontalAlignment', 'center');

== system hcu_main_dspace/RTICANMM ControllerSetup ==
  VariationInput : Inport
  Reset : Inport  Port=2
  ModelClose : Subsystem  mask(RTICANMMModelClose){}
  RTICANMMCHANNEL_TLC : S-Function  FunctionName=rticanmm_tlc_adv  Parameters=1401,1,1,0,500,'unused'  EnableBusSupport=off  mask(RTICANMMCHANNEL_TLC){}
  Variation_DTC : DataTypeConversion  SaturateOnIntegerOverflow=on  RndMeth=Zero
  sfcn : S-Function  InitFcn=rticanmm_initfcn(gcb, 'SFCNs')  FunctionName=RTICANMM_SETUP_CAN_1  EnableBusSupport=off
      mask init:
      | rticanmm_initfcn(gcb, 'SFCNs')
  wires:
  Reset/1 -> sfcn/2
  VariationInput/1 -> Variation_DTC/1
  Variation_DTC/1 -> sfcn/1

== system hcu_main_dspace/RTICANMM ControllerSetup1 ==
  VariationInput : Inport
  Reset : Inport  Port=2
  ModelClose : Subsystem  mask(RTICANMMModelClose){}
  RTICANMMCHANNEL_TLC : S-Function  FunctionName=rticanmm_tlc_adv  Parameters=1401,1,2,0,500,'unused'  EnableBusSupport=off  mask(RTICANMMCHANNEL_TLC){}
  Variation_DTC : DataTypeConversion  SaturateOnIntegerOverflow=on  RndMeth=Zero
  sfcn : S-Function  InitFcn=rticanmm_initfcn(gcb, 'SFCNs')  FunctionName=RTICANMM_SETUP_CAN_2  EnableBusSupport=off
      mask init:
      | rticanmm_initfcn(gcb, 'SFCNs')
  wires:
  Reset/1 -> sfcn/2
  VariationInput/1 -> Variation_DTC/1
  Variation_DTC/1 -> sfcn/1

== system hcu_main_dspace/RTICANMM GeneralSetup ==
  ModelClose : Subsystem  mask(RTICANMMModelClose){}
  TRC Exclusion : rtimmsu_dsrtlib/TRC Exclusion

== system hcu_main_dspace/RTICANMM MainBlock ==
  TXData : Inport
  ModelClose : Subsystem  mask(RTICANMMModelClose){}
  TRC Exclusion : rtimmsu_dsrtlib/TRC Exclusion
  TXINselector1 : BusSelector  OutputSignals=ABS2_C.BrkSw_Sta,ABS2_C.BrkSw_V,ABS2_C.VehSpeed,ABS4_C.YawRate,ABS4_C.SteerAng,ABS4_C.SteerAng_Sensor_V,ABS4_C.YawRate_V,ABS4_C.SteerAng_V,SAS1.SAS_CheckSum,SAS1.SAS_MsgCount,SAS1.SAS_OK,SAS1.SAS_CAL,SAS1.SAS_Angle,SpeedInformation.radarDeviceSpeedDirection,SpeedInformation.radarDeviceSpeed,YawRateInformation.radarDeviceYawRate
  converter : Subsystem  mask(CANnedyVector2Bus){}
      mask help: Do not change.
      mask Display: disp('Vector to\nBus')
  sfcn : S-Function  InitFcn=rticanmm_initfcn(gcb, 'SFCNs')  FunctionName=RTICANMM_MAIN_CAN_2  EnableBusSupport=off
      mask init:
      | rticanmm_initfcn(gcb, 'SFCNs')
  RX_Data : Outport
  wires:
  TXData/1 -> TXINselector1/1
  TXINselector1/1 -> sfcn/1  "<BrkSw_Sta>"
  TXINselector1/2 -> sfcn/2  "<BrkSw_V>"
  TXINselector1/3 -> sfcn/3  "<VehSpeed>"
  TXINselector1/4 -> sfcn/4  "<YawRate>"
  TXINselector1/5 -> sfcn/5  "<SteerAng>"
  TXINselector1/6 -> sfcn/6  "<SteerAng_Sensor_V>"
  TXINselector1/7 -> sfcn/7  "<YawRate_V>"
  TXINselector1/8 -> sfcn/8  "<SteerAng_V>"
  TXINselector1/9 -> sfcn/9  "<SAS_CheckSum>"
  TXINselector1/10 -> sfcn/10  "<SAS_MsgCount>"
  TXINselector1/11 -> sfcn/11  "<SAS_OK>"
  TXINselector1/12 -> sfcn/12  "<SAS_CAL>"
  TXINselector1/13 -> sfcn/13  "<SAS_Angle>"
  TXINselector1/14 -> sfcn/14  "<radarDeviceSpeedDirection>"
  TXINselector1/15 -> sfcn/15  "<radarDeviceSpeed>"
  TXINselector1/16 -> sfcn/16  "<radarDeviceYawRate>"
  converter/1(out) -> RX_Data/1
  sfcn/1 -> converter/1(in_1)
  sfcn/2 -> converter/2(in_2)
  sfcn/3 -> converter/3(in_3)
  sfcn/4 -> converter/4(in_4)
  sfcn/5 -> converter/5(in_5)
  sfcn/6 -> converter/6(in_6)
  sfcn/7 -> converter/7(in_7)
  sfcn/8 -> converter/8(in_8)
  sfcn/9 -> converter/9(in_9)
  sfcn/10 -> converter/10(in_10)
  sfcn/11 -> converter/11(in_11)
  sfcn/12 -> converter/12(in_12)
  sfcn/13 -> converter/13(in_13)
  sfcn/14 -> converter/14(in_14)
  sfcn/15 -> converter/15(in_15)
  sfcn/16 -> converter/16(in_16)
  sfcn/17 -> converter/17(in_17)
  sfcn/18 -> converter/18(in_18)
  sfcn/19 -> converter/19(in_19)
  sfcn/20 -> converter/20(in_20)
  sfcn/21 -> converter/21(in_21)
  sfcn/22 -> converter/22(in_22)
  sfcn/23 -> converter/23(in_23)
  sfcn/24 -> converter/24(in_24)
  sfcn/25 -> converter/25(in_25)
  sfcn/26 -> converter/26(in_26)
  sfcn/27 -> converter/27(in_27)
  sfcn/28 -> converter/28(in_28)
  sfcn/29 -> converter/29(in_29)
  sfcn/30 -> converter/30(in_30)
  sfcn/31 -> converter/31(in_31)
  sfcn/32 -> converter/32(in_32)
  sfcn/33 -> converter/33(in_33)
  sfcn/34 -> converter/34(in_34)
  sfcn/35 -> converter/35(in_35)
  sfcn/36 -> converter/36(in_36)
  sfcn/37 -> converter/37(in_37)
  sfcn/38 -> converter/38(in_38)
  sfcn/39 -> converter/39(in_39)
  sfcn/40 -> converter/40(in_40)
  sfcn/41 -> converter/41(in_41)
  sfcn/42 -> converter/42(in_42)
  sfcn/43 -> converter/43(in_43)
  sfcn/44 -> converter/44(in_44)
  sfcn/45 -> converter/45(in_45)
  sfcn/46 -> converter/46(in_46)
  sfcn/47 -> converter/47(in_47)
  sfcn/48 -> converter/48(in_48)
  sfcn/49 -> converter/49(in_49)
  sfcn/50 -> converter/50(in_50)
  sfcn/51 -> converter/51(in_51)
  sfcn/52 -> converter/52(in_52)
  sfcn/53 -> converter/53(in_53)
  sfcn/54 -> converter/54(in_54)
  sfcn/55 -> converter/55(in_55)
  sfcn/56 -> converter/56(in_56)
  sfcn/57 -> converter/57(in_57)
  sfcn/58 -> converter/58(in_58)
  sfcn/59 -> converter/59(in_59)
  sfcn/60 -> converter/60(in_60)
  sfcn/61 -> converter/61(in_61)
  sfcn/62 -> converter/62(in_62)
  sfcn/63 -> converter/63(in_63)
  sfcn/64 -> converter/64(in_64)
  sfcn/65 -> converter/65(in_65)
  sfcn/66 -> converter/66(in_66)
  sfcn/67 -> converter/67(in_67)
  sfcn/68 -> converter/68(in_68)
  sfcn/69 -> converter/69(in_69)
  sfcn/70 -> converter/70(in_70)
  sfcn/71 -> converter/71(in_71)
  sfcn/72 -> converter/72(in_72)
  sfcn/73 -> converter/73(in_73)
  sfcn/74 -> converter/74(in_74)
  sfcn/75 -> converter/75(in_75)
  sfcn/76 -> converter/76(in_76)
  sfcn/77 -> converter/77(in_77)
  sfcn/78 -> converter/78(in_78)
  sfcn/79 -> converter/79(in_79)
  sfcn/80 -> converter/80(in_80)
  sfcn/81 -> converter/81(in_81)
  sfcn/82 -> converter/82(in_82)
  sfcn/83 -> converter/83(in_83)
  sfcn/84 -> converter/84(in_84)
  sfcn/85 -> converter/85(in_85)
  sfcn/86 -> converter/86(in_86)
  sfcn/87 -> converter/87(in_87)
  sfcn/88 -> converter/88(in_88)
  sfcn/89 -> converter/89(in_89)
  sfcn/90 -> converter/90(in_90)
  sfcn/91 -> converter/91(in_91)
  sfcn/92 -> converter/92(in_92)
  sfcn/93 -> converter/93(in_93)
  sfcn/94 -> converter/94(in_94)
  sfcn/95 -> converter/95(in_95)
  sfcn/96 -> converter/96(in_96)
  sfcn/97 -> converter/97(in_97)
  sfcn/98 -> converter/98(in_98)
  sfcn/99 -> converter/99(in_99)
  sfcn/100 -> converter/100(in_100)
  sfcn/101 -> converter/101(in_101)
  sfcn/102 -> converter/102(in_102)
  sfcn/103 -> converter/103(in_103)
  sfcn/104 -> converter/104(in_104)
  sfcn/105 -> converter/105(in_105)
  sfcn/106 -> converter/106(in_106)
  sfcn/107 -> converter/107(in_107)
  sfcn/108 -> converter/108(in_108)
  sfcn/109 -> converter/109(in_109)
  sfcn/110 -> converter/110(in_110)
  sfcn/111 -> converter/111(in_111)
  sfcn/112 -> converter/112(in_112)
  sfcn/113 -> converter/113(in_113)
  sfcn/114 -> converter/114(in_114)
  sfcn/115 -> converter/115(in_115)
  sfcn/116 -> converter/116(in_116)
  sfcn/117 -> converter/117(in_117)
  sfcn/118 -> converter/118(in_118)
  sfcn/119 -> converter/119(in_119)
  sfcn/120 -> converter/120(in_120)
  sfcn/121 -> converter/121(in_121)
  sfcn/122 -> converter/122(in_122)
  sfcn/123 -> converter/123(in_123)
  sfcn/124 -> converter/124(in_124)
  sfcn/125 -> converter/125(in_125)
  sfcn/126 -> converter/126(in_126)
  sfcn/127 -> converter/127(in_127)
  sfcn/128 -> converter/128(in_128)
  sfcn/129 -> converter/129(in_129)
  sfcn/130 -> converter/130(in_130)
  sfcn/131 -> converter/131(in_131)
  sfcn/132 -> converter/132(in_132)
  sfcn/133 -> converter/133(in_133)
  sfcn/134 -> converter/134(in_134)
  sfcn/135 -> converter/135(in_135)
  sfcn/136 -> converter/136(in_136)
  sfcn/137 -> converter/137(in_137)
  sfcn/138 -> converter/138(in_138)
  sfcn/139 -> converter/139(in_139)
  sfcn/140 -> converter/140(in_140)
  sfcn/141 -> converter/141(in_141)
  sfcn/142 -> converter/142(in_142)
  sfcn/143 -> converter/143(in_143)
  sfcn/144 -> converter/144(in_144)
  sfcn/145 -> converter/145(in_145)
  sfcn/146 -> converter/146(in_146)
  sfcn/147 -> converter/147(in_147)
  sfcn/148 -> converter/148(in_148)
  sfcn/149 -> converter/149(in_149)
  sfcn/150 -> converter/150(in_150)
  sfcn/151 -> converter/151(in_151)
  sfcn/152 -> converter/152(in_152)
  sfcn/153 -> converter/153(in_153)
  sfcn/154 -> converter/154(in_154)
  sfcn/155 -> converter/155(in_155)
  sfcn/156 -> converter/156(in_156)
  sfcn/157 -> converter/157(in_157)
  sfcn/158 -> converter/158(in_158)
  sfcn/159 -> converter/159(in_159)
  sfcn/160 -> converter/160(in_160)
  sfcn/161 -> converter/161(in_161)
  sfcn/162 -> converter/162(in_162)
  sfcn/163 -> converter/163(in_163)
  sfcn/164 -> converter/164(in_164)
  sfcn/165 -> converter/165(in_165)
  sfcn/166 -> converter/166(in_166)
  sfcn/167 -> converter/167(in_167)
  sfcn/168 -> converter/168(in_168)
  sfcn/169 -> converter/169(in_169)
  sfcn/170 -> converter/170(in_170)
  sfcn/171 -> converter/171(in_171)
  sfcn/172 -> converter/172(in_172)
  sfcn/173 -> converter/173(in_173)
  sfcn/174 -> converter/174(in_174)
  sfcn/175 -> converter/175(in_175)
  sfcn/176 -> converter/176(in_176)
  sfcn/177 -> converter/177(in_177)
  sfcn/178 -> converter/178(in_178)
  sfcn/179 -> converter/179(in_179)
  sfcn/180 -> converter/180(in_180)
  sfcn/181 -> converter/181(in_181)
  sfcn/182 -> converter/182(in_182)
  sfcn/183 -> converter/183(in_183)
  sfcn/184 -> converter/184(in_184)
  sfcn/185 -> converter/185(in_185)
  sfcn/186 -> converter/186(in_186)
  sfcn/187 -> converter/187(in_187)
  sfcn/188 -> converter/188(in_188)
  sfcn/189 -> converter/189(in_189)
  sfcn/190 -> converter/190(in_190)
  sfcn/191 -> converter/191(in_191)
  sfcn/192 -> converter/192(in_192)
  sfcn/193 -> converter/193(in_193)
  sfcn/194 -> converter/194(in_194)
  sfcn/195 -> converter/195(in_195)
  sfcn/196 -> converter/196(in_196)
  sfcn/197 -> converter/197(in_197)
  sfcn/198 -> converter/198(in_198)
  sfcn/199 -> converter/199(in_199)
  sfcn/200 -> converter/200(in_200)
  sfcn/201 -> converter/201(in_201)
  sfcn/202 -> converter/202(in_202)
  sfcn/203 -> converter/203(in_203)
  sfcn/204 -> converter/204(in_204)
  sfcn/205 -> converter/205(in_205)
  sfcn/206 -> converter/206(in_206)
  sfcn/207 -> converter/207(in_207)
  sfcn/208 -> converter/208(in_208)
  sfcn/209 -> converter/209(in_209)
  sfcn/210 -> converter/210(in_210)
  sfcn/211 -> converter/211(in_211)
  sfcn/212 -> converter/212(in_212)
  sfcn/213 -> converter/213(in_213)
  sfcn/214 -> converter/214(in_214)
  sfcn/215 -> converter/215(in_215)
  sfcn/216 -> converter/216(in_216)
  sfcn/217 -> converter/217(in_217)
  sfcn/218 -> converter/218(in_218)
  sfcn/219 -> converter/219(in_219)
  sfcn/220 -> converter/220(in_220)
  sfcn/221 -> converter/221(in_221)
  sfcn/222 -> converter/222(in_222)
  sfcn/223 -> converter/223(in_223)
  sfcn/224 -> converter/224(in_224)
  sfcn/225 -> converter/225(in_225)
  sfcn/226 -> converter/226(in_226)
  sfcn/227 -> converter/227(in_227)
  sfcn/228 -> converter/228(in_228)
  sfcn/229 -> converter/229(in_229)
  sfcn/230 -> converter/230(in_230)
  sfcn/231 -> converter/231(in_231)
  sfcn/232 -> converter/232(in_232)
  sfcn/233 -> converter/233(in_233)
  sfcn/234 -> converter/234(in_234)
  sfcn/235 -> converter/235(in_235)
  sfcn/236 -> converter/236(in_236)
  sfcn/237 -> converter/237(in_237)
  sfcn/238 -> converter/238(in_238)
  sfcn/239 -> converter/239(in_239)
  sfcn/240 -> converter/240(in_240)
  sfcn/241 -> converter/241(in_241)
  sfcn/242 -> converter/242(in_242)
  sfcn/243 -> converter/243(in_243)
  sfcn/244 -> converter/244(in_244)
  sfcn/245 -> converter/245(in_245)
  sfcn/246 -> converter/246(in_246)
  sfcn/247 -> converter/247(in_247)
  sfcn/248 -> converter/248(in_248)
  sfcn/249 -> converter/249(in_249)
  sfcn/250 -> converter/250(in_250)
  sfcn/251 -> converter/251(in_251)
  sfcn/252 -> converter/252(in_252)
  sfcn/253 -> converter/253(in_253)
  sfcn/254 -> converter/254(in_254)
  sfcn/255 -> converter/255(in_255)
  sfcn/256 -> converter/256(in_256)
  sfcn/257 -> converter/257(in_257)
  sfcn/258 -> converter/258(in_258)
  sfcn/259 -> converter/259(in_259)
  sfcn/260 -> converter/260(in_260)
  sfcn/261 -> converter/261(in_261)
  sfcn/262 -> converter/262(in_262)
  sfcn/263 -> converter/263(in_263)
  sfcn/264 -> converter/264(in_264)
  sfcn/265 -> converter/265(in_265)
  sfcn/266 -> converter/266(in_266)
  sfcn/267 -> converter/267(in_267)
  sfcn/268 -> converter/268(in_268)
  sfcn/269 -> converter/269(in_269)
  sfcn/270 -> converter/270(in_270)
  sfcn/271 -> converter/271(in_271)
  sfcn/272 -> converter/272(in_272)
  sfcn/273 -> converter/273(in_273)
  sfcn/274 -> converter/274(in_274)
  sfcn/275 -> converter/275(in_275)
  sfcn/276 -> converter/276(in_276)
  sfcn/277 -> converter/277(in_277)
  sfcn/278 -> converter/278(in_278)
  sfcn/279 -> converter/279(in_279)
  sfcn/280 -> converter/280(in_280)
  sfcn/281 -> converter/281(in_281)
  sfcn/282 -> converter/282(in_282)
  sfcn/283 -> converter/283(in_283)
  sfcn/284 -> converter/284(in_284)
  sfcn/285 -> converter/285(in_285)
  sfcn/286 -> converter/286(in_286)
  sfcn/287 -> converter/287(in_287)
  sfcn/288 -> converter/288(in_288)
  sfcn/289 -> converter/289(in_289)
  sfcn/290 -> converter/290(in_290)
  sfcn/291 -> converter/291(in_291)
  sfcn/292 -> converter/292(in_292)
  sfcn/293 -> converter/293(in_293)
  sfcn/294 -> converter/294(in_294)
  sfcn/295 -> converter/295(in_295)
  sfcn/296 -> converter/296(in_296)
  sfcn/297 -> converter/297(in_297)
  sfcn/298 -> converter/298(in_298)
  sfcn/299 -> converter/299(in_299)
  sfcn/300 -> converter/300(in_300)
  sfcn/301 -> converter/301(in_301)
  sfcn/302 -> converter/302(in_302)
  sfcn/303 -> converter/303(in_303)
  sfcn/304 -> converter/304(in_304)
  sfcn/305 -> converter/305(in_305)
  sfcn/306 -> converter/306(in_306)
  sfcn/307 -> converter/307(in_307)
  sfcn/308 -> converter/308(in_308)
  sfcn/309 -> converter/309(in_309)
  sfcn/310 -> converter/310(in_310)
  sfcn/311 -> converter/311(in_311)
  sfcn/312 -> converter/312(in_312)
  sfcn/313 -> converter/313(in_313)
  sfcn/314 -> converter/314(in_314)
  sfcn/315 -> converter/315(in_315)
  sfcn/316 -> converter/316(in_316)
  sfcn/317 -> converter/317(in_317)
  sfcn/318 -> converter/318(in_318)
  sfcn/319 -> converter/319(in_319)
  sfcn/320 -> converter/320(in_320)
  sfcn/321 -> converter/321(in_321)
  sfcn/322 -> converter/322(in_322)
  sfcn/323 -> converter/323(in_323)
  sfcn/324 -> converter/324(in_324)
  sfcn/325 -> converter/325(in_325)
  sfcn/326 -> converter/326(in_326)
  sfcn/327 -> converter/327(in_327)
  sfcn/328 -> converter/328(in_328)
  sfcn/329 -> converter/329(in_329)
  sfcn/330 -> converter/330(in_330)
  sfcn/331 -> converter/331(in_331)
  sfcn/332 -> converter/332(in_332)
  sfcn/333 -> converter/333(in_333)
  sfcn/334 -> converter/334(in_334)
